simulink model "Acrobot"  (R2022b)
settings: Solver=VariableStepAuto  StartTime=0.0  StopTime=40  FixedStep=1/30  RelTol=1e-3
values from neighbouring files (symbols this model uses):
  F = lqr(Alin, Blin, Q, R)    [startup.m]
  g = 9.81    [startup.m]
  I1 = 1/3*m1*L1^2    (= 0.021951)    [startup.m]
  I2 = 1/3*m2*L2^2    (= 0.813)    [startup.m]
  L1 = 0.3    [startup.m]
  Lc1 = L1/2    (= 0.15)    [startup.m]
  Lc2 = L2/2    (= 0.5)    [startup.m]
  m1 = L1*(0.03)*(0.03)*rho_aluminum    (= 0.7317)    [startup.m]
  m2 = L2*(0.03)*(0.03)*rho_aluminum    (= 2.439)    [startup.m]
  q1_0 = deg2rad(-100)    [startup.m]
  q2_0 = deg2rad(-45)    [startup.m]
settings Model: Creator=logan  LastModifiedBy=logan

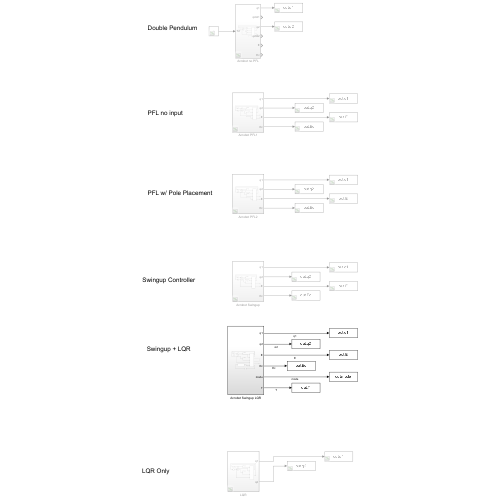
[thumbnail: Simulink's stored preview of the top-level diagram]
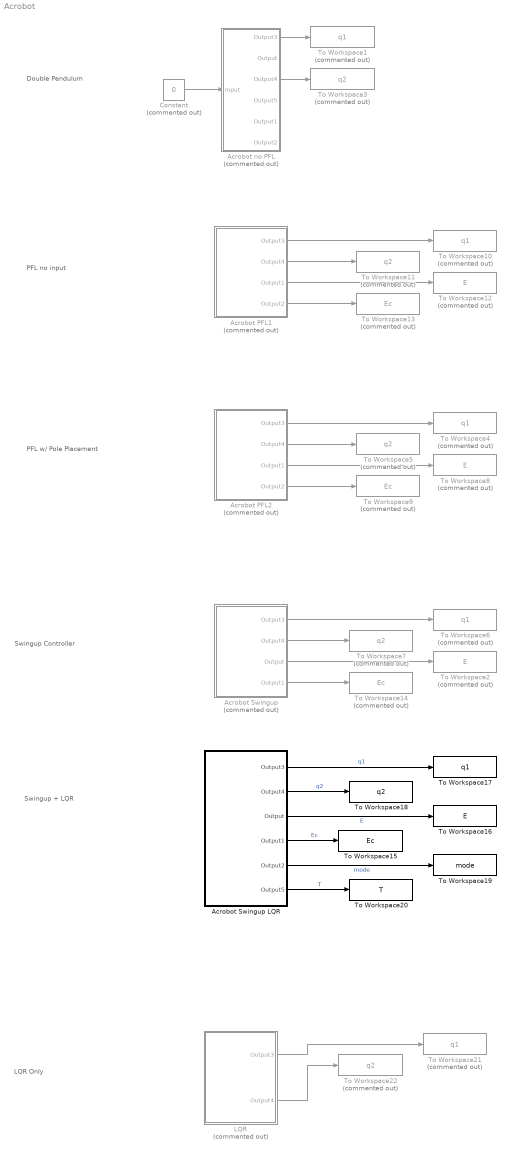
== system Acrobot ==
  note: Double Pendulum
  note: PFL no input
  note: PFL w/ Pole Placement
  note: Swingup Controller
  note: Swingup + LQR
  note: LQR Only
  Acrobot PFL1 : Subsystem  Commented=on
  Acrobot PFL2 : Subsystem  Commented=on
  Acrobot Swingup : Subsystem  Commented=on
  Acrobot Swingup LQR : Subsystem
  Acrobot no PFL : Subsystem  Commented=on
  Constant : Constant  Commented=on  Value=0
  LQR : Subsystem  Commented=on
  To Workspace{1,4,6,10,21} (5 alike) : ToWorkspace  Commented=on  VariableName=q1  SaveFormat=Timeseries  SampleTime=-1
  To Workspace{3,5,7,11,22} (5 alike) : ToWorkspace  Commented=on  VariableName=q2  SaveFormat=Timeseries  SampleTime=-1
  To Workspace12 : ToWorkspace  Commented=on  VariableName=E  SaveFormat=Timeseries  SampleTime=-1
  To Workspace13 : ToWorkspace  Commented=on  VariableName=Ec  SaveFormat=Timeseries  SampleTime=-1
  To Workspace14 : ToWorkspace  Commented=on  VariableName=Ec  SaveFormat=Timeseries  SampleTime=-1
  To Workspace15 : ToWorkspace  VariableName=Ec  SaveFormat=Timeseries  SampleTime=-1
  To Workspace16 : ToWorkspace  VariableName=E  SaveFormat=Timeseries  SampleTime=-1
  To Workspace17 : ToWorkspace  VariableName=q1  SaveFormat=Timeseries  SampleTime=-1
  To Workspace18 : ToWorkspace  VariableName=q2  SaveFormat=Timeseries  SampleTime=-1
  To Workspace19 : ToWorkspace  VariableName=mode  SaveFormat=Timeseries  SampleTime=-1
  To Workspace2 : ToWorkspace  Commented=on  VariableName=E  SaveFormat=Timeseries  SampleTime=-1
  To Workspace20 : ToWorkspace  VariableName=T  SaveFormat=Timeseries  SampleTime=-1
  To Workspace8 : ToWorkspace  Commented=on  VariableName=E  SaveFormat=Timeseries  SampleTime=-1
  To Workspace9 : ToWorkspace  Commented=on  VariableName=Ec  SaveFormat=Timeseries  SampleTime=-1
  wires:
  Acrobot no PFL/1(Output3) -> To Workspace1/1
  Acrobot no PFL/3(Output4) -> To Workspace3/1
  Constant/1 -> Acrobot no PFL/1(Input)
  Acrobot PFL2/2(Output4) -> To Workspace5/1
  Acrobot PFL2/1(Output3) -> To Workspace4/1
  Acrobot Swingup/2(Output4) -> To Workspace7/1
  Acrobot Swingup/1(Output3) -> To Workspace6/1
  Acrobot PFL2/3(Output1) -> To Workspace8/1
  Acrobot PFL2/4(Output2) -> To Workspace9/1
  Acrobot PFL1/3(Output1) -> To Workspace12/1
  Acrobot PFL1/4(Output2) -> To Workspace13/1
  Acrobot PFL1/2(Output4) -> To Workspace11/1
  Acrobot PFL1/1(Output3) -> To Workspace10/1
  Acrobot Swingup/3(Output) -> To Workspace2/1
  Acrobot Swingup/4(Output1) -> To Workspace14/1
  Acrobot Swingup LQR/3(Output) -> To Workspace16/1  "E"
  Acrobot Swingup LQR/2(Output4) -> To Workspace18/1  "q2"
  Acrobot Swingup LQR/4(Output1) -> To Workspace15/1  "Ec"
  Acrobot Swingup LQR/1(Output3) -> To Workspace17/1  "q1"
  LQR/1(Output3) -> To Workspace21/1
  LQR/2(Output4) -> To Workspace22/1
  Acrobot Swingup LQR/5(Output2) -> To Workspace19/1  "mode"
  Acrobot Swingup LQR/6(Output5) -> To Workspace20/1  "T"

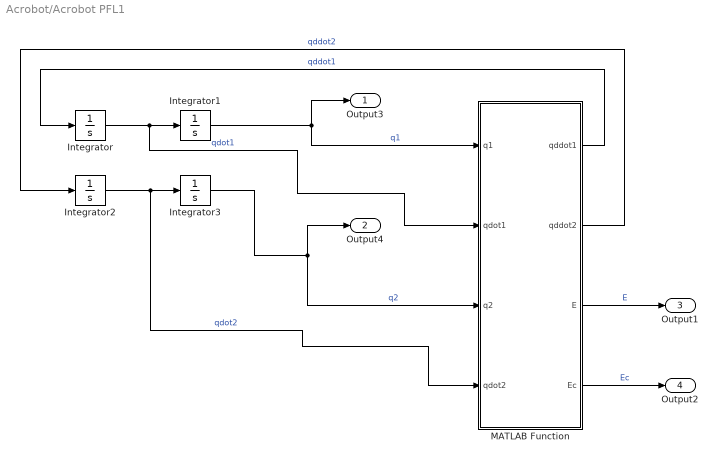
== system Acrobot/Acrobot PFL1 ==
  Integrator : Integrator
  Integrator1 : Integrator  InitialCondition=q1_0
  Integrator2 : Integrator
  Integrator3 : Integrator  InitialCondition=q2_0
  MATLAB Function : MATLAB Function  TreatAsAtomicUnit=on
  Output3 : Outport
  Output4 : Outport  Port=2
  Output1 : Outport  Port=3
  Output2 : Outport  Port=4
  wires:
  Integrator/1 -> MATLAB Function/2(qdot1), Integrator1/1  "qdot1"
  Integrator1/1 -> Output3/1, MATLAB Function/1(q1)  "q1"
  MATLAB Function/3(E) -> Output1/1  "E"
  MATLAB Function/4(Ec) -> Output2/1  "Ec"
  Integrator2/1 -> MATLAB Function/4(qdot2), Integrator3/1  "qdot2"
  MATLAB Function/2(qddot2) -> Integrator2/1  "qddot2"
  Integrator3/1 -> Output4/1, MATLAB Function/3(q2)  "q2"
  MATLAB Function/1(qddot1) -> Integrator/1  "qddot1"

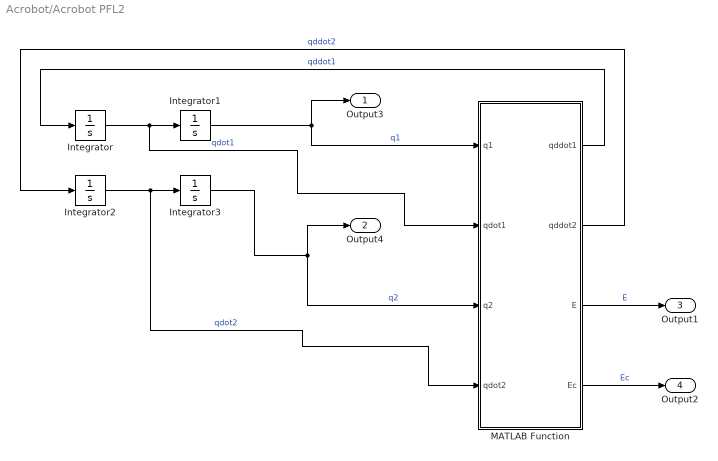
== system Acrobot/Acrobot PFL2 ==
  Integrator : Integrator
  Integrator1 : Integrator  InitialCondition=q1_0
  Integrator2 : Integrator
  Integrator3 : Integrator  InitialCondition=q2_0
  MATLAB Function : MATLAB Function  TreatAsAtomicUnit=on
  Output3 : Outport
  Output4 : Outport  Port=2
  Output1 : Outport  Port=3
  Output2 : Outport  Port=4
  wires:
  Integrator/1 -> MATLAB Function/2(qdot1), Integrator1/1  "qdot1"
  Integrator1/1 -> Output3/1, MATLAB Function/1(q1)  "q1"
  MATLAB Function/3(E) -> Output1/1  "E"
  MATLAB Function/4(Ec) -> Output2/1  "Ec"
  Integrator2/1 -> MATLAB Function/4(qdot2), Integrator3/1  "qdot2"
  MATLAB Function/2(qddot2) -> Integrator2/1  "qddot2"
  Integrator3/1 -> Output4/1, MATLAB Function/3(q2)  "q2"
  MATLAB Function/1(qddot1) -> Integrator/1  "qddot1"

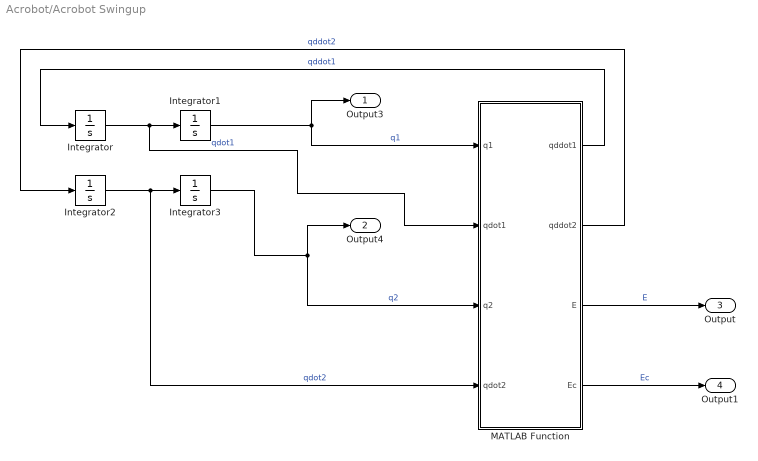
== system Acrobot/Acrobot Swingup ==
  Integrator : Integrator
  Integrator1 : Integrator  InitialCondition=q1_0
  Integrator2 : Integrator
  Integrator3 : Integrator  InitialCondition=q2_0
  MATLAB Function : MATLAB Function  TreatAsAtomicUnit=on
  Output3 : Outport
  Output4 : Outport  Port=2
  Output : Outport  Port=3
  Output1 : Outport  Port=4
  wires:
  Integrator/1 -> MATLAB Function/2(qdot1), Integrator1/1  "qdot1"
  Integrator1/1 -> Output3/1, MATLAB Function/1(q1)  "q1"
  Integrator2/1 -> MATLAB Function/4(qdot2), Integrator3/1  "qdot2"
  MATLAB Function/2(qddot2) -> Integrator2/1  "qddot2"
  Integrator3/1 -> Output4/1, MATLAB Function/3(q2)  "q2"
  MATLAB Function/1(qddot1) -> Integrator/1  "qddot1"
  MATLAB Function/3(E) -> Output/1  "E"
  MATLAB Function/4(Ec) -> Output1/1  "Ec"

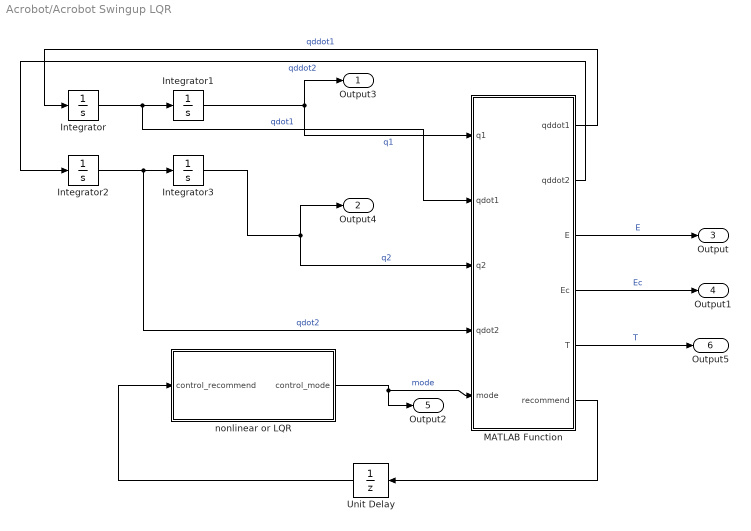
== system Acrobot/Acrobot Swingup LQR ==
  Integrator : Integrator
  Integrator1 : Integrator  InitialCondition=q1_0
  Integrator2 : Integrator
  Integrator3 : Integrator  InitialCondition=q2_0
  MATLAB Function : MATLAB Function  TreatAsAtomicUnit=on
  Unit Delay : UnitDelay  SampleTime=1/30  HasFrameUpgradeWarning=on
  nonlinear or LQR : Stateflow chart  TreatAsAtomicUnit=on
  Output3 : Outport
  Output4 : Outport  Port=2
  Output : Outport  Port=3
  Output1 : Outport  Port=4
  Output2 : Outport  Port=5
  Output5 : Outport  Port=6
  wires:
  Integrator/1 -> MATLAB Function/2(qdot1), Integrator1/1  "qdot1"
  Integrator1/1 -> Output3/1, MATLAB Function/1(q1)  "q1"
  Integrator2/1 -> MATLAB Function/4(qdot2), Integrator3/1  "qdot2"
  MATLAB Function/2(qddot2) -> Integrator2/1  "qddot2"
  Integrator3/1 -> Output4/1, MATLAB Function/3(q2)  "q2"
  MATLAB Function/1(qddot1) -> Integrator/1  "qddot1"
  MATLAB Function/3(E) -> Output/1  "E"
  MATLAB Function/4(Ec) -> Output1/1  "Ec"
  nonlinear or LQR/1(control_mode) -> Output2/1, MATLAB Function/5(mode)  "mode"
  MATLAB Function/6(recommend) -> Unit Delay/1
  Unit Delay/1 -> nonlinear or LQR/1(control_recommend)
  MATLAB Function/5(T) -> Output5/1  "T"

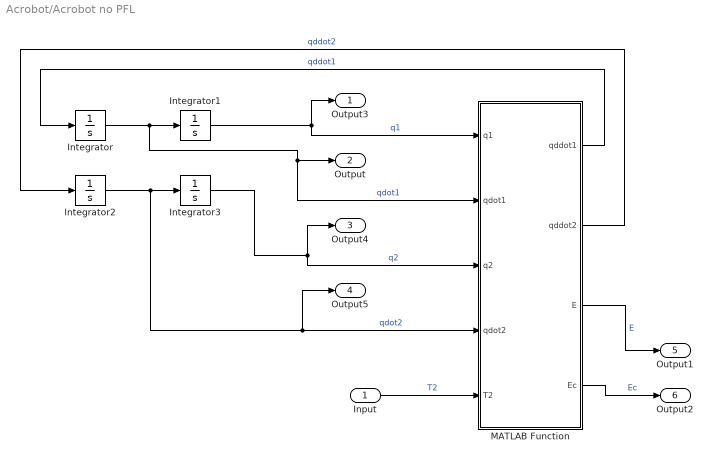
== system Acrobot/Acrobot no PFL ==
  Input : Inport
  Integrator : Integrator
  Integrator1 : Integrator  InitialCondition=q1_0
  Integrator2 : Integrator
  Integrator3 : Integrator  InitialCondition=q2_0
  MATLAB Function : MATLAB Function  TreatAsAtomicUnit=on
  Output3 : Outport
  Output : Outport  Port=2
  Output4 : Outport  Port=3
  Output5 : Outport  Port=4
  Output1 : Outport  Port=5
  Output2 : Outport  Port=6
  wires:
  Integrator2/1 -> Output5/1, MATLAB Function/4(qdot2), Integrator3/1  "qdot2"
  Integrator/1 -> Output/1, MATLAB Function/2(qdot1), Integrator1/1  "qdot1"
  Integrator3/1 -> Output4/1, MATLAB Function/3(q2)  "q2"
  MATLAB Function/2(qddot2) -> Integrator2/1  "qddot2"
  MATLAB Function/1(qddot1) -> Integrator/1  "qddot1"
  Integrator1/1 -> Output3/1, MATLAB Function/1(q1)  "q1"
  MATLAB Function/3(E) -> Output1/1  "E"
  MATLAB Function/4(Ec) -> Output2/1  "Ec"
  Input/1 -> MATLAB Function/5(T2)  "T2"

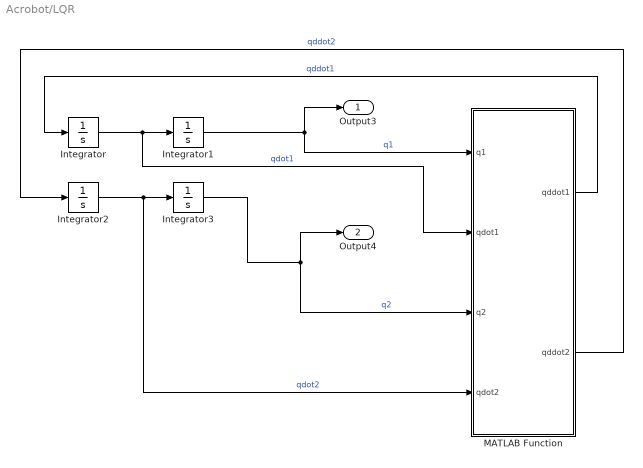
== system Acrobot/LQR ==
  Integrator : Integrator
  Integrator1 : Integrator  InitialCondition=pi/2 + 0.1
  Integrator2 : Integrator
  Integrator3 : Integrator  InitialCondition=-0.2
  MATLAB Function : MATLAB Function  TreatAsAtomicUnit=on
  Output3 : Outport
  Output4 : Outport  Port=2
  wires:
  Integrator/1 -> MATLAB Function/2(qdot1), Integrator1/1  "qdot1"
  Integrator1/1 -> Output3/1, MATLAB Function/1(q1)  "q1"
  Integrator2/1 -> MATLAB Function/4(qdot2), Integrator3/1  "qdot2"
  MATLAB Function/2(qddot2) -> Integrator2/1  "qddot2"
  Integrator3/1 -> Output4/1, MATLAB Function/3(q2)  "q2"
  MATLAB Function/1(qddot1) -> Integrator/1  "qddot1"

== matlab function Acrobot/Acrobot PFL1/MATLAB Function ==
  data: q1 input; qdot1 input; q2 input; qdot2 input; qddot1 output; qddot2 output; g parameter; I2 parameter; Lc2 parameter; m2 parameter; I1 parameter; Lc1 parameter; L1 parameter; m1 parameter; E output; Ec output
function [qddot1,qddot2,E,Ec] = ...
    EoM(q1,qdot1,q2,qdot2, g, I2, Lc2, m2, I1, Lc1, L1, m1)

m11 = m1*Lc1^2 + m2*(L1^2 + Lc2^2 + 2*L1*Lc2*cos(q2)) + I1 + I2;
m12 = m2*(Lc2^2 + L1*Lc2*cos(q2)) + I2;
m22 = m2*Lc2^2 + I2;

h1 = -m2*L1*Lc2*sin(q2)*qdot2^2 - 2*m2*L1*Lc2*sin(q2)*qdot2*qdot1;
phi1 = (m1*Lc1+m2*L1)*g*cos(q1) + m2*Lc2*g*cos(q1+q2);

% equations of motion (PFL)
u = 0;
qddot2 = u;
qddot1 = -1/m11*(m12*u + h1 + phi1);

% energy calculations
yc1 = Lc1*sin(q1);
yc2 = L1*sin(q1) + Lc2*sin(q1+q2);

K = 0.5*m11*qdot1^2 + m12*qdot1*qdot2 + 0.5*m22*qdot2^2;
P = g*(m1*yc1 + m2*yc2);
E = K + P;
Ec = g*(m1*Lc1 + m2*(L1+Lc2)); % upright potential energy

== matlab function Acrobot/Acrobot Swingup/MATLAB Function ==
  data: q1 input; qdot1 input; q2 input; qdot2 input; qddot1 output; qddot2 output; g parameter; I2 parameter; Lc2 parameter; m2 parameter; I1 parameter; Lc1 parameter; L1 parameter; m1 parameter; E output; Ec output
function [qddot1,qddot2,E,Ec] = ...
    EoM(q1,qdot1,q2,qdot2,g, I2, Lc2, m2, I1, Lc1, L1, m1)

m11 = m1*Lc1^2 + m2*(L1^2 + Lc2^2 + 2*L1*Lc2*cos(q2)) + I1 + I2;
m12 = m2*(Lc2^2 + L1*Lc2*cos(q2)) + I2;
m22 = m2*Lc2^2 + I2;

h1 = -m2*L1*Lc2*sin(q2)*qdot2^2 - 2*m2*L1*Lc2*sin(q2)*qdot2*qdot1;
phi1 = (m1*Lc1+m2*L1)*g*cos(q1) + m2*Lc2*g*cos(q1+q2);

% energy calculations
yc1 = Lc1*sin(q1);
yc2 = L1*sin(q1) + Lc2*sin(q1+q2);K = 0.5*m11*qdot1^2 + m12*qdot1*qdot2 + 0.5*m22*qdot2^2;
P = g*(m1*yc1 + m2*yc2);
E = K + P;
Ec = g*(m1*Lc1 + m2*(L1+Lc2)); % upright potential energy

% equations of motion (PFL)
% with pole placement
% and nonlinear swingup control
k2 = 10;
k1 = 21;

u_bar = (Ec-E)*qdot1;
sat_ubar = min(10, max(-10, u_bar));
% sat_ubar = u_bar;

u = sat_ubar - k2*qdot2 - k1*q2;
qddot2 = u;
qddot1 = -1/m11*(m12*u + h1 + phi1);

== matlab function Acrobot/LQR/MATLAB Function ==
  data: q1 input; qdot1 input; q2 input; qdot2 input; qddot1 output; qddot2 output; g parameter; I2 parameter; Lc2 parameter; m2 parameter; I1 parameter; Lc1 parameter; L1 parameter; m1 parameter; F parameter
function [qddot1,qddot2] = ...
    EoM(q1,qdot1,q2,qdot2,g, I2, Lc2, m2, I1, Lc1, L1, m1, F)

m11 = m1*Lc1^2 + m2*(L1^2 + Lc2^2 + 2*L1*Lc2*cos(q2)) + I1 + I2;
m12 = m2*(Lc2^2 + L1*Lc2*cos(q2)) + I2;
m22 = m2*Lc2^2 + I2;

h1 = -m2*L1*Lc2*sin(q2)*qdot2^2 - 2*m2*L1*Lc2*sin(q2)*qdot2*qdot1;
h2 = m2*L1*Lc2*sin(q2)*qdot1^2;

phi1 = (m1*Lc1+m2*L1)*g*cos(q1) + m2*Lc2*g*cos(q1+q2);
phi2 = m2*Lc2*g*cos(q1+q2);

m22_bar = m22 - m12^2/m11;
h2_bar = h2 - m12*h1/m11;
phi2_bar = phi2 - m12*phi1/m11;

% LQR (accounting for non-zero set point)
q1_adj = wrapToPi(q1);
q2_adj = wrapToPi(q2);
T_lqr = -F*[q1_adj-pi/2; q2_adj; qdot1; qdot2];

% dynamics
qddot2 = 1/m22_bar*(T_lqr - h2_bar - phi2_bar);
qddot1 = -1/m11*(m12*qddot2 + h1 + phi1);

== stateflow chart Acrobot/Acrobot Swingup LQR/nonlinear or LQR ==
  state nonlinear
    control_mode=1;
  state LQR
    control_mode=2;
  (default) -> nonlinear
  nonlinear -> LQR : [control_recommend==2]
  data: control_recommend input; control_mode output

== matlab function Acrobot/Acrobot Swingup LQR/MATLAB Function ==
  data: q1 input; qdot1 input; q2 input; qdot2 input; mode input; qddot1 output; qddot2 output; g parameter; I2 parameter; Lc2 parameter; m2 parameter; I1 parameter; Lc1 parameter; L1 parameter; m1 parameter; E output; Ec output; T output; F parameter; recommend output
function [qddot1,qddot2,E,Ec,T,recommend] = ...
    EoM(q1,qdot1,q2,qdot2,mode,g,I2,Lc2,m2,I1,Lc1,L1,m1,F)

% equations of motion
m11 = m1*Lc1^2 + m2*(L1^2 + Lc2^2 + 2*L1*Lc2*cos(q2)) + I1 + I2;
m12 = m2*(Lc2^2 + L1*Lc2*cos(q2)) + I2;
m22 = m2*Lc2^2 + I2;

h1 = -m2*L1*Lc2*sin(q2)*qdot2^2 - 2*m2*L1*Lc2*sin(q2)*qdot2*qdot1;
h2 = m2*L1*Lc2*sin(q2)*qdot1^2;

phi1 = (m1*Lc1+m2*L1)*g*cos(q1) + m2*Lc2*g*cos(q1+q2);
phi2 = m2*Lc2*g*cos(q1+q2);

m22_bar = m22 - m12^2/m11;
h2_bar = h2 - m12*h1/m11;
phi2_bar = phi2 - m12*phi1/m11;

% energy calculations
yc1 = Lc1*sin(q1);
yc2 = L1*sin(q1) + Lc2*sin(q1+q2);
K = 0.5*m11*qdot1^2 + m12*qdot1*qdot2 + 0.5*m22*qdot2^2;
P = g*(m1*yc1 + m2*yc2);
E = K + P;
Ec = g*(m1*Lc1 + m2*(L1+Lc2)); % upright potential energy

% equations of motion (PFL)
% with pole placement
% and nonlinear swingup control
k2 = 10;
k1 = 21;

u_bar = (Ec-E)*qdot1;
u_nonlinear = u_bar - k2*qdot2 - k1*q2;
T_nonlinear = m22_bar*u_nonlinear + h2_bar + phi2_bar;

% LQR (accounting for non-zero set point)
z1 = wrapToPi(q1)-pi/2;
z2 = wrapToPi(q2);
T_lqr = -F*[z1; z2; qdot1; qdot2];

% dynamics
if mode == 1
    T = T_nonlinear;
else
    T = T_lqr;
end

% saturation
T = min(25, max(-25, T));
qddot2 = 1/m22_bar*(T - h2_bar - phi2_bar);
qddot1 = -1/m11*(m12*qddot2 + h1 + phi1);


% starts in nonlinear mode, switches to LQR at the right moment
% does not switch back to nonlinear mode once we are in LQR
if abs(z1) < deg2rad(5)
    recommend = 2; % LQR
else
    recommend = 1; % nonlinear
end

== matlab function Acrobot/Acrobot no PFL/MATLAB Function ==
  data: q1 input; qdot1 input; q2 input; qdot2 input; qddot1 output; qddot2 output; T2 input; g parameter; I2 parameter; Lc2 parameter; m2 parameter; I1 parameter; Lc1 parameter; L1 parameter; m1 parameter; E output; Ec output
function [qddot1,qddot2,E,Ec] = ...
    EoM(q1,qdot1,q2,qdot2,T2, g, I2, Lc2, m2, I1, Lc1, L1, m1)

m11 = m1*Lc1^2 + m2*(L1^2 + Lc2^2 + 2*L1*Lc2*cos(q2)) + I1 + I2;
m12 = m2*(Lc2^2 + L1*Lc2*cos(q2)) + I2;
m22 = m2*Lc2^2 + I2;

h1 = -m2*L1*Lc2*sin(q2)*qdot2^2 - 2*m2*L1*Lc2*sin(q2)*qdot2*qdot1;
h2 = m2*L1*Lc2*sin(q2)*qdot1^2;

phi1 = (m1*Lc1+m2*L1)*g*cos(q1) + m2*Lc2*g*cos(q1+q2);
phi2 = m2*Lc2*g*cos(q1+q2);

m22_bar = m22 - m12^2/m11;
h2_bar = h2 - m12*h1/m11;
phi2_bar = phi2 - m12*phi1/m11;

% equations of motion
qddot2 = 1/m22_bar*(T2 - h2_bar - phi2_bar);
qddot1 = -1/m11*(m12*qddot2 + h1 + phi1);

% energy calculations
yc1 = Lc1*sin(q1);
yc2 = L1*sin(q1) + Lc2*sin(q1+q2);

K = 0.5*m11*qdot1^2 + m12*qdot1*qdot2 + 0.5*m22*qdot2^2;
P = g*(m1*yc1 + m2*yc2);
E = K + P;
Ec = g*(m1*Lc1 + m2*(L1+Lc2)); % upright potential energy

== matlab function Acrobot/Acrobot PFL2/MATLAB Function ==
  data: q1 input; qdot1 input; q2 input; qdot2 input; qddot1 output; qddot2 output; g parameter; I2 parameter; Lc2 parameter; m2 parameter; I1 parameter; Lc1 parameter; L1 parameter; m1 parameter; E output; Ec output
function [qddot1,qddot2,E,Ec] = ...
    EoM(q1,qdot1,q2,qdot2, g, I2, Lc2, m2, I1, Lc1, L1, m1)

m11 = m1*Lc1^2 + m2*(L1^2 + Lc2^2 + 2*L1*Lc2*cos(q2)) + I1 + I2;
m12 = m2*(Lc2^2 + L1*Lc2*cos(q2)) + I2;
m22 = m2*Lc2^2 + I2;

h1 = -m2*L1*Lc2*sin(q2)*qdot2^2 - 2*m2*L1*Lc2*sin(q2)*qdot2*qdot1;
phi1 = (m1*Lc1+m2*L1)*g*cos(q1) + m2*Lc2*g*cos(q1+q2);

% equations of motion (PFL)
% with pole placement at (s+3)(s+7)
k1 = 21;
k2 = 10;
qddot2 = - k2*qdot2 - k1*q2;
qddot1 = -1/m11*(m12*qddot2 + h1 + phi1);

% energy calculations
yc1 = Lc1*sin(q1);
yc2 = L1*sin(q1) + Lc2*sin(q1+q2);

K = 0.5*m11*qdot1^2 + m12*qdot1*qdot2 + 0.5*m22*qdot2^2;
P = g*(m1*yc1 + m2*yc2);
E = K + P;
Ec = g*(m1*Lc1 + m2*(L1+Lc2)); % upright potential energy
